simulink model "PlantNL"  (R2015b)
settings: Solver=VariableStepAuto  StartTime=0.0  StopTime=10.0  RelTol=1e-3
settings Model: Creator=gnardelli  LastModifiedBy=gnardelli

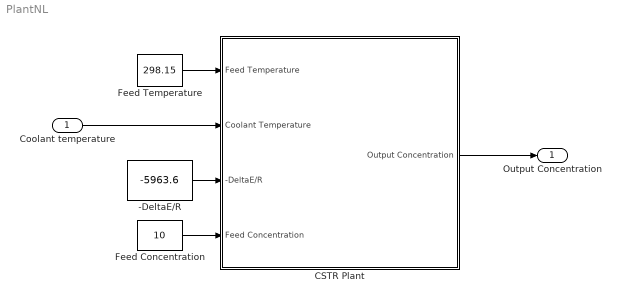
== system PlantNL ==
  Coolant temperature : Inport
  -DeltaE/R : Constant  Value=-5963.6  SampleTime=0
  CSTR Plant : Subsystem
  Feed Concentration : Constant  Value=10  SampleTime=0
  Feed Temperature : Constant  Value=298.15  SampleTime=0
  Output Concentration : Outport
  wires:
  Feed Temperature/1 -> CSTR Plant/1(Feed Temperature)
  -DeltaE/R/1 -> CSTR Plant/3(-DeltaE/R)
  Feed Concentration/1 -> CSTR Plant/4(Feed Concentration)
  CSTR Plant/1(Output Concentration) -> Output Concentration/1
  Coolant temperature/1 -> CSTR Plant/2(Coolant Temperature)

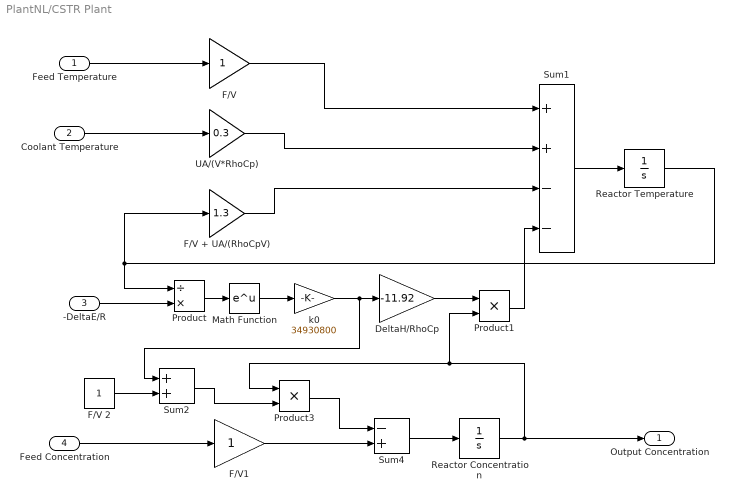
== system PlantNL/CSTR Plant ==
  Feed Temperature : Inport
  Coolant Temperature : Inport  Port=2
  -DeltaE/R : Inport  Port=3
  Feed Concentration : Inport  Port=4
  DeltaH/RhoCp : Gain  Gain=-11.92  SaturateOnIntegerOverflow=on  OutDataTypeStr=Inherit: Same as input  ParamDataTypeStr=Inherit: Same as input
  F/V : Gain  SaturateOnIntegerOverflow=on  OutDataTypeStr=Inherit: Same as input  ParamDataTypeStr=Inherit: Same as input
  F/V + UA/(RhoCpV) : Gain  Gain=1.3  SaturateOnIntegerOverflow=on  OutDataTypeStr=Inherit: Same as input  ParamDataTypeStr=Inherit: Same as input
  F/V 2 : Constant  SampleTime=0
  F/V1 : Gain  SaturateOnIntegerOverflow=on  OutDataTypeStr=Inherit: Same as input  ParamDataTypeStr=Inherit: Same as input
  Math Function : Math  SaturateOnIntegerOverflow=on
  Product : Product  Inputs=/*  SaturateOnIntegerOverflow=on  RndMeth=Zero  InputSameDT=on  OutDataTypeStr=Inherit: Same as first input
  Product1 : Product  SaturateOnIntegerOverflow=on  RndMeth=Zero  InputSameDT=on  OutDataTypeStr=Inherit: Same as first input
  Product3 : Product  SaturateOnIntegerOverflow=on  RndMeth=Zero  InputSameDT=on  OutDataTypeStr=Inherit: Same as first input
  Reactor Concentration : Integrator  InitialCondition=5  LimitOutput=on  LowerSaturationLimit=0
  Reactor Temperature : Integrator  InitialCondition=300  LimitOutput=on  LowerSaturationLimit=0
  Sum1 : Sum  Inputs=++--  SaturateOnIntegerOverflow=on  InputSameDT=on  OutDataTypeStr=Inherit: Same as first input
  Sum2 : Sum  SaturateOnIntegerOverflow=on  InputSameDT=on  OutDataTypeStr=Inherit: Same as first input
  Sum4 : Sum  Inputs=-+  SaturateOnIntegerOverflow=on  InputSameDT=on  OutDataTypeStr=Inherit: Same as first input
  UA/(V*RhoCp) : Gain  Gain=0.3  SaturateOnIntegerOverflow=on  OutDataTypeStr=Inherit: Same as input  ParamDataTypeStr=Inherit: Same as input
  k0 : Gain  Gain=34930800  SaturateOnIntegerOverflow=on  OutDataTypeStr=Inherit: Same as input  ParamDataTypeStr=Inherit: Same as input
  Output Concentration : Outport
  wires:
  Sum2/1 -> Product3/2
  Coolant Temperature/1 -> UA/(V*RhoCp)/1
  Feed Concentration/1 -> F/V1/1
  Feed Temperature/1 -> F/V/1
  F/V1/1 -> Sum4/2
  F/V 2/1 -> Sum2/2
  Reactor Concentration/1 -> Output Concentration/1, Product1/2, Product3/1
  Sum4/1 -> Reactor Concentration/1
  Product3/1 -> Sum4/1
  -DeltaE/R/1 -> Product/2
  k0/1 -> Sum2/1, DeltaH/RhoCp/1
  Product1/1 -> Sum1/4
  DeltaH/RhoCp/1 -> Product1/1
  Math Function/1 -> k0/1
  Product/1 -> Math Function/1
  F/V + UA/(RhoCpV)/1 -> Sum1/3
  UA/(V*RhoCp)/1 -> Sum1/2
  Reactor Temperature/1 -> F/V + UA/(RhoCpV)/1, Product/1
  Sum1/1 -> Reactor Temperature/1
  F/V/1 -> Sum1/1
